simulink model "single_sat_attitude"  (R2018a)
settings: Solver=ode1  StartTime=0.0  StopTime=10.0  FixedStep=1/100  RelTol=1e-3
undefined symbols (not defined in the file or in its folder): Earth, h_init, hdmax, hmax, IAU, init, Kd, km, Kp, NRLMSISE_time_fromJD, q_init, s, wbn_init, WGS84
libraries: aerolibtransform2 x9, aerolibutil x6, sharedtransform x4, simulink x4, aerolibcelestial x3, vrlib x3, aerolibgravity2 x2, aerolibconvert2 x2, sharedutil x2, aerolibatmos2 x1
(part 2 of 2)

== system single_sat_attitude/Plant/Sun Torque and Force ==
  quat_in_body : Inport  PortDimensions=4
  sunBlocked : Inport  Port=2  OutDataTypeStr=boolean  PortDimensions=1
  sattosun_plant_eci : Inport  Port=3  PortDimensions=3
  4th real to 1st real : Subsystem
  Constant : Constant  Value=comtocops
  Constant1 : Constant  Value=unitnormals
  Constant2 : Constant  Value=areas
  Constant4 : Constant  Value=rss
  Constant5 : Constant  Value=rds
  Gain : Gain  Gain=-1
  Quaternion Rotation : aerolibutil/Quaternion Rotation
  Switch : Switch  Criteria=u2 ~= 0
  Zero : Constant  Value=0
  pressureTorque : MATLAB Function  TreatAsAtomicUnit=on
  solar pressure constant : Constant  Value=4.644E-6
  sunT_out_body : Outport  Unit=N*m  PortDimensions=3
  sunF_out_body : Outport  Port=2  Unit=N  PortDimensions=3
  wires:
  pressureTorque/2(torque) -> sunT_out_body/1
  Constant4/1 -> pressureTorque/6(rss)
  Constant/1 -> pressureTorque/5(comtocops)
  Constant1/1 -> pressureTorque/4(unitnormals)
  Constant2/1 -> pressureTorque/3(areas)
  sattosun_plant_eci/1 -> Quaternion Rotation/2
  Gain/1 -> pressureTorque/2(unitvelocity)
  Quaternion Rotation/1 -> Gain/1
  pressureTorque/1(force) -> sunF_out_body/1
  Constant5/1 -> pressureTorque/7(rds)
  sunBlocked/1 -> Switch/2
  Zero/1 -> Switch/1
  solar pressure constant/1 -> Switch/3
  Switch/1 -> pressureTorque/1(pressure)
  quat_in_body/1 -> 4th real to 1st real/1(qin)
  4th real to 1st real/1(qout) -> Quaternion Rotation/1

== system single_sat_attitude/Plant/circular_orbit ==
  time_elapsed : Inport  Unit=s  PortDimensions=1
  Gain1 : Gain  Gain=W
  Gain2 : Gain  Gain=PPERP
  Gain3 : Gain  Gain=P
  Gain4 : Gain  Gain=-P
  Gain5 : Gain  Gain=PPERP
  Gain6 : Gain  Gain=W
  Sin : Trigonometry
  Sin1 : Trigonometry  Operator=cos
  Sum2 : Sum  Inputs=+|+
  Sum5 : Sum  Inputs=+|+
  r_eci : Outport  Unit=m  PortDimensions=3
  v_eci : Outport  Port=2  Unit=m/s  PortDimensions=3
  wires:
  Gain5/1 -> Sum5/2
  Sum2/1 -> r_eci/1
  Gain2/1 -> Sum2/1
  Gain3/1 -> Sum2/2
  Gain4/1 -> Sum5/1
  Gain1/1 -> Sin/1, Sin1/1
  Sin1/1 -> Gain5/1, Gain3/1
  time_elapsed/1 -> Gain1/1
  Sum5/1 -> Gain6/1
  Sin/1 -> Gain4/1, Gain2/1
  Gain6/1 -> v_eci/1

== system single_sat_attitude/Sensor Model/Gyro ==
  note: Gyro: LSM6DS33
  body_w : Inport  Unit=rad/s
  DCM to translate from body to sensor : Constant  Value=init.IMU0_DCM_BODY
  Data Type Conversion : DataTypeConversion  OutDataTypeStr=int16  RndMeth=Round  SaturateOnIntegerOverflow=on
  Matrix Multiply1 : Product  Multiplication=Matrix(*)
  Random Number : RandomNumber  Mean=init.IMU0_G_TYOFF  Variance=init.IMU0_G_RMS.^2  SampleTime=1.0/init.IMU0_G_ODR
  Saturation : Saturate  UpperLimit=init.IMU0_G_FS  LowerLimit=-init.IMU0_G_FS
  Sum : Sum  Inputs=|++
  Zero-Order Hold : ZeroOrderHold  SampleTime=1.0/init.IMU0_G_ODR
  sensitivity : Gain  Gain=init.IMU0_G_GN
  sensor_w : Outport  OutDataTypeStr=int16
  wires:
  DCM to translate from body to sensor/1 -> Matrix Multiply1/1
  body_w/1 -> Matrix Multiply1/2
  sensitivity/1 -> Data Type Conversion/1
  Data Type Conversion/1 -> sensor_w/1
  Random Number/1 -> Sum/2
  Sum/1 -> sensitivity/1
  Saturation/1 -> Sum/1
  Zero-Order Hold/1 -> Saturation/1
  Matrix Multiply1/1 -> Zero-Order Hold/1

== system single_sat_attitude/Sensor Model/Magnetometer ==
  note: Magnetometer: LIS3MDL
      | see the data sheet for more details
  Magnetic_Field_body : Inport  Unit=nT
  DCM to translate from body to sensor : Constant  Value=init.IMU0_DCM_BODY
  Data Type Conversion : DataTypeConversion  OutDataTypeStr=int16  RndMeth=Round
  Matrix Multiply2 : Product  Multiplication=Matrix(*)
  Random Number : RandomNumber  Mean=-init.IMU0_MAG_ZGAUSS  Variance=init.IMU0_MAG_RMS.^2  SampleTime=1.0/init.IMU0_MAG_ODR
  Sum : Sum  Inputs=|++
  Zero-Order Hold : ZeroOrderHold  SampleTime=1.0/init.IMU0_MAG_ODR
  sensitivity : Gain  Gain=init.IMU0_MAG_GN
  Magxyz : Outport  OutDataTypeStr=int16
  wires:
  Data Type Conversion/1 -> Magxyz/1
  sensitivity/1 -> Data Type Conversion/1
  Matrix Multiply2/1 -> Zero-Order Hold/1
  Zero-Order Hold/1 -> Sum/1
  Sum/1 -> sensitivity/1
  Random Number/1 -> Sum/2
  Magnetic_Field_body/1 -> Matrix Multiply2/2
  DCM to translate from body to sensor/1 -> Matrix Multiply2/1

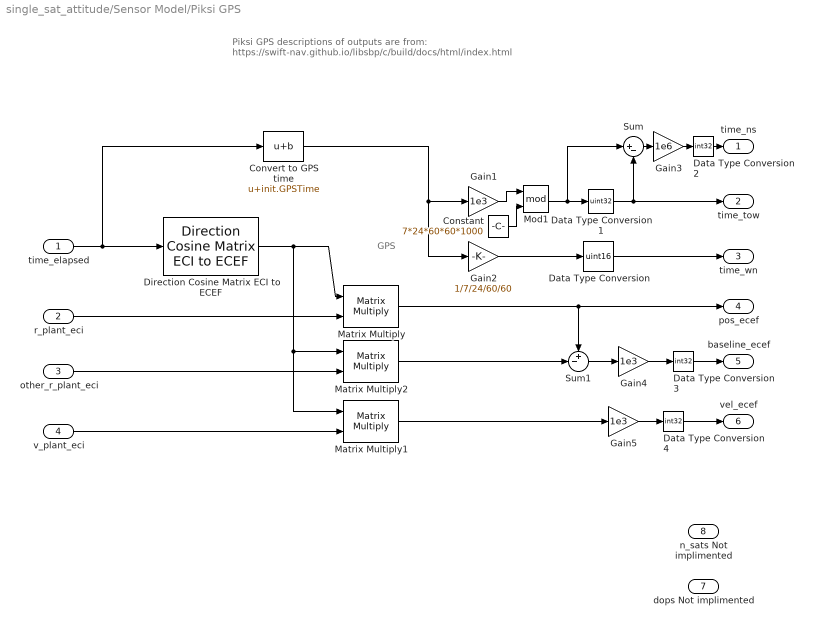
== system single_sat_attitude/Sensor Model/Piksi GPS ==
  note: Piksi GPS
      |
      | descriptions of outputs are from:
      | https://swift-nav.github.io/libsbp/c/build/docs/html/index.html
  note: GPS
  time_elapsed : Inport  Unit=s
  r_plant_eci : Inport  Port=2  Unit=m
  other_r_plant_eci : Inport  Port=3  Unit=m
  v_plant_eci : Inport  Port=4  Unit=m/s
  Constant : Constant  Value=7*24*60*60*1000
  Convert to GPS time : Bias  Bias=init.GPSTime
  Data Type Conversion : DataTypeConversion  OutDataTypeStr=uint16
  Data Type Conversion1 : DataTypeConversion  OutDataTypeStr=uint32  RndMeth=Round
  Data Type Conversion2 : DataTypeConversion  OutDataTypeStr=int32  RndMeth=Simplest
  Data Type Conversion3 : DataTypeConversion  OutDataTypeStr=int32  RndMeth=Simplest
  Data Type Conversion4 : DataTypeConversion  OutDataTypeStr=int32  RndMeth=Simplest
  Direction Cosine Matrix ECI to ECEF : aerolibtransform2/Direction Cosine Matrix ECI to ECEF  red=IAU-2000/2006  year=init.year  month=October  day=20  hour=init.hour  min=init.min  sec=init.sec  deltaT=Sec  errorflag=Error  extraparamflag=off
      settings: AttributesFormatString=%<red>  SourceProductName=Aerospace Blockset  SourceProductBaseCode=AE
  Gain1 : Gain  Gain=1e3
  Gain2 : Gain  Gain=1/7/24/60/60
  Gain3 : Gain  Gain=1e6
  Gain4 : Gain  Gain=1e3
  Gain5 : Gain  Gain=1e3
  Matrix Multiply : Product  Multiplication=Matrix(*)  OutDataTypeStr=double
  Matrix Multiply1 : Product  Multiplication=Matrix(*)
  Matrix Multiply2 : Product  Multiplication=Matrix(*)  OutDataTypeStr=double
  Mod1 : Math  Operator=mod  SaturateOnIntegerOverflow=on
  Sum : Sum  Inputs=|+-
  Sum1 : Sum  Inputs=+-|
  time_ns : Outport  OutMin=[-500000]  OutMax=[500000]  OutDataTypeStr=int32  Unit=ns  SampleTime=1/init.GPS_ODR
      settings: AttributesFormatString=Nanosecond residual of millisecond-rounded TOW
  time_tow : Outport  Port=2  OutMin=[0]  OutDataTypeStr=uint32  Unit=ms  SampleTime=1/init.GPS_ODR
      settings: AttributesFormatString=GPS time of week rounded to the nearest millisecond
  time_wn : Outport  Port=3  OutDataTypeStr=uint16  Unit=weeks  SampleTime=1/init.GPS_ODR
      settings: AttributesFormatString=GPS week number
  pos_ecef : Outport  Port=4  OutDataTypeStr=double  Unit=m  SampleTime=1/init.GPS_ODR
      settings: AttributesFormatString=absolute Earth Centered Earth Fixed (ECEF) coordinates
  baseline_ecef : Outport  Description=Dilution of Precision p,t  Port=5  OutDataTypeStr=int32  Unit=mm  SampleTime=1/init.GPS_ODR
      settings: AttributesFormatString=relative vector distance from the base station to the rover receiver.
  vel_ecef : Outport  Port=6  OutDataTypeStr=int32  Unit=mm/s  SampleTime=1/init.GPS_ODR
      settings: AttributesFormatString=velocity in Earth Centered Earth Fixed (ECEF) coordinates.
  dops Not implimented : Outport  Port=7  SampleTime=1/init.GPS_ODR
      settings: AttributesFormatString=|
      | Dilution of Precision p,t
      | describes the effect of navigation satellite geometry on positional measurement precision.
  n_sats Not implimented : Outport  Port=8  OutDataTypeStr=uint8  SampleTime=1/init.GPS_ODR
      settings: AttributesFormatString=Number of satellites used in solution.
  wires:
  Direction Cosine Matrix ECI to ECEF/1 -> Matrix Multiply1/1, Matrix Multiply2/1, Matrix Multiply/1
  time_elapsed/1 -> Direction Cosine Matrix ECI to ECEF/1, Convert to GPS time/1
  v_plant_eci/1 -> Matrix Multiply1/2
  Matrix Multiply/1 -> Sum1/1, pos_ecef/1
  r_plant_eci/1 -> Matrix Multiply/2
  Convert to GPS time/1 -> Gain2/1, Gain1/1
  Gain1/1 -> Mod1/1
  Data Type Conversion1/1 -> Sum/2, time_tow/1
  Sum/1 -> Gain3/1
  other_r_plant_eci/1 -> Matrix Multiply2/2
  Matrix Multiply2/1 -> Sum1/2
  Constant/1 -> Mod1/2
  Mod1/1 -> Data Type Conversion1/1, Sum/1
  Gain2/1 -> Data Type Conversion/1
  Data Type Conversion/1 -> time_wn/1
  Gain3/1 -> Data Type Conversion2/1
  Data Type Conversion2/1 -> time_ns/1
  Gain4/1 -> Data Type Conversion3/1
  Sum1/1 -> Gain4/1
  Data Type Conversion3/1 -> baseline_ecef/1
  Matrix Multiply1/1 -> Gain5/1
  Gain5/1 -> Data Type Conversion4/1
  Data Type Conversion4/1 -> vel_ecef/1

== system single_sat_attitude/Sensor Model/quat to DCM ==
  e0 e1 e2 e3 : Inport
  Demux : Demux
  Gain1 : Gain  Gain=2  SaturateOnIntegerOverflow=on  OutDataTypeStr=Inherit: Same as input  ParamDataTypeStr=Inherit: Same as input
  Gain2 : Gain  Gain=2  SaturateOnIntegerOverflow=on  OutDataTypeStr=Inherit: Same as input  ParamDataTypeStr=Inherit: Same as input
  Matrix Gain : Gain  Gain=eye(3,3)  SaturateOnIntegerOverflow=on  OutDataTypeStr=Inherit: Same as input  ParamDataTypeStr=Inherit: Same as input
  Mux : Mux  Inputs=3
  Product : Product  SaturateOnIntegerOverflow=on  InputSameDT=on  OutDataTypeStr=Inherit: Same as first input
  Product1 : Product  SaturateOnIntegerOverflow=on  InputSameDT=on  OutDataTypeStr=Inherit: Same as first input
  Subsystem : Subsystem
      mask Display: disp('3x3 cross matrix')
  Sum1 : Sum  Inputs=|+-  SaturateOnIntegerOverflow=on  InputSameDT=on  OutDataTypeStr=Inherit: Same as first input
  Sum8 : Sum  Inputs=|+-+  SaturateOnIntegerOverflow=on  InputSameDT=on  OutDataTypeStr=Inherit: Same as first input
  T1 : Math  Operator=transpose  SaturateOnIntegerOverflow=on
  T2 : Math  Operator=transpose  SaturateOnIntegerOverflow=on
  qTq : Product  Multiplication=Matrix(*)  SaturateOnIntegerOverflow=on  InputSameDT=on  OutDataTypeStr=Inherit: Same as first input
  qqT : Product  Multiplication=Matrix(*)  SaturateOnIntegerOverflow=on  InputSameDT=on  OutDataTypeStr=Inherit: Same as first input
  DCM : Outport  InitialOutput=0
  wires:
  Sum8/1 -> DCM/1
  e0 e1 e2 e3/1 -> Demux/1
  Demux/1 -> Mux/1
  Demux/2 -> Mux/2
  Demux/3 -> Mux/3
  Demux/4 -> Product/2, Product1/1, Product1/2
  Mux/1 -> T1/1, qqT/1, Subsystem/1(In1), T2/1, qTq/2
  Product/1 -> Gain1/1
  T1/1 -> qqT/2
  qqT/1 -> Gain2/1
  Gain2/1 -> Sum8/1
  Gain1/1 -> Sum8/2
  Product1/1 -> Sum1/1
  T2/1 -> qTq/1
  qTq/1 -> Sum1/2
  Sum1/1 -> Matrix Gain/1
  Matrix Gain/1 -> Sum8/3
  Subsystem/1(Out1) -> Product/1

== system single_sat_attitude/Actuator Model1/Rigid Body with Momentum Actuators and energy dissipation/Cross1 ==
  A : Inport  PortDimensions=3
  B : Inport  Port=2  PortDimensions=3
  Mux4 : Mux  Inputs=3
  Product{,1..5} (6 alike) : Product  SaturateOnIntegerOverflow=on  InputSameDT=on  OutDataTypeStr=Inherit: Same as first input
  Sum : Sum  Inputs=+-  SaturateOnIntegerOverflow=on  InputSameDT=on  OutDataTypeStr=Inherit: Same as first input
  Sum1 : Sum  Inputs=+-  SaturateOnIntegerOverflow=on  InputSameDT=on  OutDataTypeStr=Inherit: Same as first input
  Sum2 : Sum  Inputs=+-  SaturateOnIntegerOverflow=on  InputSameDT=on  OutDataTypeStr=Inherit: Same as first input
  demux2 : Demux  Outputs=3
  demux3 : Demux  Outputs=3
  AxB : Outport  InitialOutput=0
  wires:
  Mux4/1 -> AxB/1
  Sum2/1 -> Mux4/3
  Sum1/1 -> Mux4/2
  Sum/1 -> Mux4/1
  Product5/1 -> Sum2/2
  Product4/1 -> Sum2/1
  Product3/1 -> Sum1/2
  Product2/1 -> Sum1/1
  Product1/1 -> Sum/2
  Product/1 -> Sum/1
  demux3/1 -> Product5/2, Product2/2
  demux2/2 -> Product5/1, Product/1
  demux3/2 -> Product4/2, Product1/2
  demux2/1 -> Product4/1, Product3/1
  demux3/3 -> Product3/2, Product/2
  demux2/3 -> Product2/1, Product1/1
  B/1 -> demux3/1
  A/1 -> demux2/1

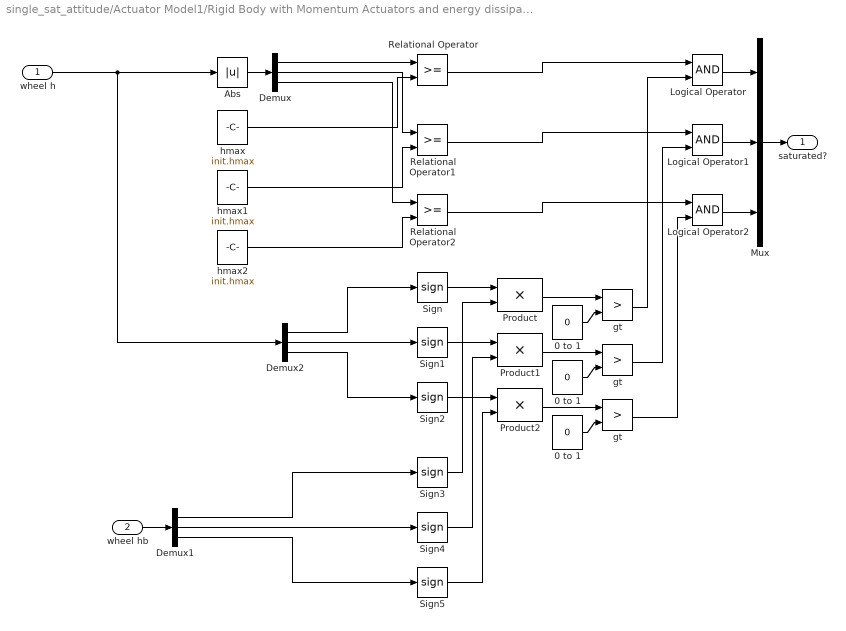
== system single_sat_attitude/Actuator Model1/Rigid Body with Momentum Actuators and energy dissipation/max rate check ==
  wheel h : Inport
  wheel hb : Inport  Port=2
  0 to 1 : Constant  Value=0  VectorParams1D=off
  "0 to 1 " : Constant  Value=0  VectorParams1D=off
  "0 to 1  " : Constant  Value=0  VectorParams1D=off
  Abs : Abs  SaturateOnIntegerOverflow=on
  Demux : Demux  Outputs=3
  Demux1 : Demux  Outputs=3
  Demux2 : Demux  Outputs=3
  Logical Operator : Logic
  Logical Operator1 : Logic
  Logical Operator2 : Logic
  Mux : Mux  Inputs=3
  Product : Product  SaturateOnIntegerOverflow=on  InputSameDT=on  OutDataTypeStr=Inherit: Same as first input
  Product1 : Product  SaturateOnIntegerOverflow=on  InputSameDT=on  OutDataTypeStr=Inherit: Same as first input
  Product2 : Product  SaturateOnIntegerOverflow=on  InputSameDT=on  OutDataTypeStr=Inherit: Same as first input
  Relational Operator : RelationalOperator  RndMeth=Nearest  InputSameDT=on
  Relational Operator1 : RelationalOperator  RndMeth=Nearest  InputSameDT=on
  Relational Operator2 : RelationalOperator  RndMeth=Nearest  InputSameDT=on
  Sign{,1..5} (6 alike) : Signum
  gt : RelationalOperator  Operator=>  RndMeth=Nearest  InputSameDT=on
  "gt " : RelationalOperator  Operator=>  RndMeth=Nearest  InputSameDT=on
  "gt  " : RelationalOperator  Operator=>  RndMeth=Nearest  InputSameDT=on
  hmax : Constant  Value=init.hmax  VectorParams1D=off
  hmax1 : Constant  Value=init.hmax  VectorParams1D=off
  hmax2 : Constant  Value=init.hmax  VectorParams1D=off
  saturated? : Outport
  wires:
  Abs/1 -> Demux/1
  Demux/1 -> Relational Operator/1
  Demux/2 -> Relational Operator1/1
  Demux/3 -> Relational Operator2/1
  hmax/1 -> Relational Operator/2
  hmax1/1 -> Relational Operator1/2
  hmax2/1 -> Relational Operator2/2
  wheel h/1 -> Abs/1, Demux2/1
  Mux/1 -> saturated?/1
  wheel hb/1 -> Demux1/1
  Demux1/1 -> Sign3/1
  Demux1/2 -> Sign4/1
  Demux1/3 -> Sign5/1
  Sign/1 -> Product/1
  Sign3/1 -> Product/2
  Sign1/1 -> Product1/1
  Sign4/1 -> Product1/2
  Sign2/1 -> Product2/1
  Sign5/1 -> Product2/2
  0 to 1/1 -> gt/2
  Product/1 -> gt/1
  "0 to 1 "/1 -> "gt "/2
  Product1/1 -> "gt "/1
  "0 to 1  "/1 -> "gt  "/2
  Product2/1 -> "gt  "/1
  Logical Operator/1 -> Mux/1
  Logical Operator1/1 -> Mux/2
  Logical Operator2/1 -> Mux/3
  Relational Operator/1 -> Logical Operator/1
  Relational Operator1/1 -> Logical Operator1/1
  Relational Operator2/1 -> Logical Operator2/1
  gt/1 -> Logical Operator/2
  "gt "/1 -> Logical Operator1/2
  "gt  "/1 -> Logical Operator2/2
  Demux2/1 -> Sign/1
  Demux2/2 -> Sign1/1
  Demux2/3 -> Sign2/1

== system single_sat_attitude/Actuator Model1/Rigid Body with Momentum Actuators and energy dissipation/quat to DCM ==
  e0 e1 e2 e3 : Inport
  Demux : Demux
  Gain1 : Gain  Gain=2  SaturateOnIntegerOverflow=on  OutDataTypeStr=Inherit: Same as input  ParamDataTypeStr=Inherit: Same as input
  Gain2 : Gain  Gain=2  SaturateOnIntegerOverflow=on  OutDataTypeStr=Inherit: Same as input  ParamDataTypeStr=Inherit: Same as input
  Matrix Gain : Gain  Gain=eye(3,3)  SaturateOnIntegerOverflow=on  OutDataTypeStr=Inherit: Same as input  ParamDataTypeStr=Inherit: Same as input
  Mux : Mux  Inputs=3
  Product : Product  SaturateOnIntegerOverflow=on  InputSameDT=on  OutDataTypeStr=Inherit: Same as first input
  Product1 : Product  SaturateOnIntegerOverflow=on  InputSameDT=on  OutDataTypeStr=Inherit: Same as first input
  Subsystem : Subsystem
      mask Display: disp('3x3 cross matrix')
  Sum1 : Sum  Inputs=|+-  SaturateOnIntegerOverflow=on  InputSameDT=on  OutDataTypeStr=Inherit: Same as first input
  Sum8 : Sum  Inputs=|+-+  SaturateOnIntegerOverflow=on  InputSameDT=on  OutDataTypeStr=Inherit: Same as first input
  T1 : Math  Operator=transpose  SaturateOnIntegerOverflow=on
  T2 : Math  Operator=transpose  SaturateOnIntegerOverflow=on
  qTq : Product  Multiplication=Matrix(*)  SaturateOnIntegerOverflow=on  InputSameDT=on  OutDataTypeStr=Inherit: Same as first input
  qqT : Product  Multiplication=Matrix(*)  SaturateOnIntegerOverflow=on  InputSameDT=on  OutDataTypeStr=Inherit: Same as first input
  DCM : Outport  InitialOutput=0
  wires:
  Subsystem/1(Out1) -> Product/1
  Matrix Gain/1 -> Sum8/3
  Sum1/1 -> Matrix Gain/1
  qTq/1 -> Sum1/2
  T2/1 -> qTq/1
  Product1/1 -> Sum1/1
  Gain1/1 -> Sum8/2
  Gain2/1 -> Sum8/1
  qqT/1 -> Gain2/1
  T1/1 -> qqT/2
  Product/1 -> Gain1/1
  Mux/1 -> qTq/2, T2/1, qqT/1, T1/1, Subsystem/1(In1)
  Demux/4 -> Product1/2, Product1/1, Product/2
  Demux/3 -> Mux/3
  Demux/2 -> Mux/2
  Demux/1 -> Mux/1
  e0 e1 e2 e3/1 -> Demux/1
  Sum8/1 -> DCM/1

== system single_sat_attitude/Actuator Model1/Rigid Body with Momentum Actuators and energy dissipation/quat to DCM1 ==
  e0 e1 e2 e3 : Inport
  Demux : Demux
  Gain1 : Gain  Gain=2  SaturateOnIntegerOverflow=on  OutDataTypeStr=Inherit: Same as input  ParamDataTypeStr=Inherit: Same as input
  Gain2 : Gain  Gain=2  SaturateOnIntegerOverflow=on  OutDataTypeStr=Inherit: Same as input  ParamDataTypeStr=Inherit: Same as input
  Matrix Gain : Gain  Gain=eye(3,3)  SaturateOnIntegerOverflow=on  OutDataTypeStr=Inherit: Same as input  ParamDataTypeStr=Inherit: Same as input
  Mux : Mux  Inputs=3
  Product : Product  SaturateOnIntegerOverflow=on  InputSameDT=on  OutDataTypeStr=Inherit: Same as first input
  Product1 : Product  SaturateOnIntegerOverflow=on  InputSameDT=on  OutDataTypeStr=Inherit: Same as first input
  Subsystem : Subsystem
      mask Display: disp('3x3 cross matrix')
  Sum1 : Sum  Inputs=|+-  SaturateOnIntegerOverflow=on  InputSameDT=on  OutDataTypeStr=Inherit: Same as first input
  Sum8 : Sum  Inputs=|+-+  SaturateOnIntegerOverflow=on  InputSameDT=on  OutDataTypeStr=Inherit: Same as first input
  T1 : Math  Operator=transpose  SaturateOnIntegerOverflow=on
  T2 : Math  Operator=transpose  SaturateOnIntegerOverflow=on
  qTq : Product  Multiplication=Matrix(*)  SaturateOnIntegerOverflow=on  InputSameDT=on  OutDataTypeStr=Inherit: Same as first input
  qqT : Product  Multiplication=Matrix(*)  SaturateOnIntegerOverflow=on  InputSameDT=on  OutDataTypeStr=Inherit: Same as first input
  DCM : Outport  InitialOutput=0
  wires:
  Subsystem/1(Out1) -> Product/1
  Matrix Gain/1 -> Sum8/3
  Sum1/1 -> Matrix Gain/1
  qTq/1 -> Sum1/2
  T2/1 -> qTq/1
  Product1/1 -> Sum1/1
  Gain1/1 -> Sum8/2
  Gain2/1 -> Sum8/1
  qqT/1 -> Gain2/1
  T1/1 -> qqT/2
  Product/1 -> Gain1/1
  Mux/1 -> qTq/2, T2/1, qqT/1, T1/1, Subsystem/1(In1)
  Demux/4 -> Product1/2, Product1/1, Product/2
  Demux/3 -> Mux/3
  Demux/2 -> Mux/2
  Demux/1 -> Mux/1
  e0 e1 e2 e3/1 -> Demux/1
  Sum8/1 -> DCM/1

== system single_sat_attitude/Attitude Determination/Attitude Determination/Generate reference vectors from Ephemeris and Magnetic Field Model ==
  note: geodetic LLA
  time_elapsed : Inport
  r_cs_sensor_eci : Inport  Port=2
  Add : Sum  Inputs=+-
  DecimalYearIncrement : Subsystem
  Demux : Demux  Outputs=3
  ECI Position to LLA : aerolibtransform2/ECI Position to LLA  red=IAU-2000/2006  year=init.year  month=October  day=20  hour=init.hour  min=init.min  sec=init.sec  deltaT=Sec  errorflag=Error  extraparamflag=off  eunits=Metric (MKS)  earthmodel=WGS84  flat=1/298.257223563  eqradius=6378137
      settings: AttributesFormatString=%<red>  SourceProductName=Aerospace Blockset  SourceProductBaseCode=AE
  International Geomagnetic Reference Field 12 : aerolibgravity2/International Geomagnetic Reference Field 12  units=Metric (MKS)  time_in=on  month=January  day=1  year=2020  action=None  sv_out=off
      settings: SourceProductName=Aerospace Blockset  SourceProductBaseCode=AE
  Julian Date : Subsystem
  Planetary Ephemeris : aerolibcelestial/Planetary Ephemeris  kmflag=km,km/s  epochflag=Julian date  de=DE430  nCenter=Earth  nTarget=Sun  errorflag=Error  velflag=off
      settings: SourceProductName=Aerospace Blockset  SourceProductBaseCode=AE
  r_Sun2cs_ref_eci : Outport
  r_MagField_ref_eci : Outport  Port=2
  wires:
  Julian Date/1(Julian Date) -> Planetary Ephemeris/1
  Planetary Ephemeris/1 -> Add/1
  Demux/1 -> International Geomagnetic Reference Field 12/2
  International Geomagnetic Reference Field 12/1 -> r_MagField_ref_eci/1
  ECI Position to LLA/1 -> Demux/1
  Demux/3 -> International Geomagnetic Reference Field 12/1
  Add/1 -> r_Sun2cs_ref_eci/1
  DecimalYearIncrement/1(DecimalYear) -> International Geomagnetic Reference Field 12/4
  r_cs_sensor_eci/1 -> Add/2, ECI Position to LLA/1
  time_elapsed/1 -> DecimalYearIncrement/1(clock_sec), ECI Position to LLA/2, Julian Date/1(deltaT)
  Demux/2 -> International Geomagnetic Reference Field 12/3

== system single_sat_attitude/Attitude Determination/Attitude Determination/Subsystem ==
  r_Sun2cs_ref_eci : Inport
  r_MagField_ref_eci : Inport  Port=2
  r_Sun2cs_sensor_body : Inport  Port=3
  r_MagField_sensor_body : Inport  Port=4
  MATLAB Function : MATLAB Function  TreatAsAtomicUnit=on
  quat_body_calc : Outport
  wires:
  r_Sun2cs_ref_eci/1 -> MATLAB Function/1(N_sun)
  r_MagField_ref_eci/1 -> MATLAB Function/2(N_mag)
  r_Sun2cs_sensor_body/1 -> MATLAB Function/3(B_sun)
  r_MagField_sensor_body/1 -> MATLAB Function/4(B_mag)
  MATLAB Function/1(q_triad) -> quat_body_calc/1

== system single_sat_attitude/Controller/Free Rigid Body with Momentum Actuators2/Cross ==
  A : Inport
  B : Inport  Port=2
  Mux4 : Mux  Inputs=3
  Product{,1..5} (6 alike) : Product  SaturateOnIntegerOverflow=on  InputSameDT=on  OutDataTypeStr=Inherit: Same as first input
  Sum : Sum  Inputs=+-  SaturateOnIntegerOverflow=on  InputSameDT=on  OutDataTypeStr=Inherit: Same as first input
  Sum1 : Sum  Inputs=+-  SaturateOnIntegerOverflow=on  InputSameDT=on  OutDataTypeStr=Inherit: Same as first input
  Sum2 : Sum  Inputs=+-  SaturateOnIntegerOverflow=on  InputSameDT=on  OutDataTypeStr=Inherit: Same as first input
  demux2 : Demux  Outputs=3
  demux3 : Demux  Outputs=3
  AxB : Outport  InitialOutput=0
  wires:
  Mux4/1 -> AxB/1
  Sum2/1 -> Mux4/3
  Sum1/1 -> Mux4/2
  Sum/1 -> Mux4/1
  Product5/1 -> Sum2/2
  Product4/1 -> Sum2/1
  Product3/1 -> Sum1/2
  Product2/1 -> Sum1/1
  Product1/1 -> Sum/2
  Product/1 -> Sum/1
  demux3/1 -> Product5/2, Product2/2
  demux2/2 -> Product5/1, Product/1
  demux3/2 -> Product4/2, Product1/2
  demux2/1 -> Product4/1, Product3/1
  demux3/3 -> Product3/2, Product/2
  demux2/3 -> Product2/1, Product1/1
  B/1 -> demux3/1
  A/1 -> demux2/1

== system single_sat_attitude/Controller/Free Rigid Body with Momentum Actuators2/Quaternion Integration ==
  w_Body : Inport
  Integrator1 : Integrator  InitialCondition=q_init
  q_normalize : Subsystem
  qderiv : Subsystem
  q_I_Body : Outport
  wires:
  qderiv/1(qd) -> Integrator1/1
  Integrator1/1 -> q_normalize/1(q_in)
  q_normalize/1(q_out) -> q_I_Body/1, qderiv/2(q)
  w_Body/1 -> qderiv/1(w)

== system single_sat_attitude/Controller/Free Rigid Body with Momentum Actuators2/RWA Saturation Model (Maxon EC 32 Flat 15W 24V) ==
  hb_com : Inport
  Demux : Demux  Outputs=3
  Demux2 : Demux  Outputs=3
  Max Torque : Saturate  UpperLimit=hdmax  LowerLimit=-hdmax
  Mux : Mux  Inputs=3
  Scope : Scope
  Switch : Switch  Threshold=0.5  SaturateOnIntegerOverflow=on  InputSameDT=on
  Switch1 : Switch  Threshold=0.5  SaturateOnIntegerOverflow=on  InputSameDT=on
  Switch2 : Switch  Threshold=0.5  SaturateOnIntegerOverflow=on  InputSameDT=on
  "hb -> h" : Integrator  InitialCondition=h_init
  max rate check : Subsystem
  no torque : Constant  Value=0
  hb_act : Outport
  h_act : Outport  Port=2
  wires:
  Switch2/1 -> Mux/3
  Switch1/1 -> Mux/2
  Demux2/3 -> Switch2/2
  Switch/1 -> Mux/1
  no torque/1 -> Switch/1, Switch1/1, Switch2/1
  Demux2/1 -> Switch/2
  Mux/1 -> Scope/1, hb_act/1, "hb -> h"/1
  hb_com/1 -> Max Torque/1
  Demux2/2 -> Switch1/2
  Demux/2 -> Switch1/3
  Demux/1 -> Switch/3
  "hb -> h"/1 -> h_act/1, max rate check/1(wheel h)
  Max Torque/1 -> Demux/1, max rate check/2(wheel hb)
  Demux/3 -> Switch2/3
  max rate check/1(saturated?) -> Demux2/1

== system single_sat_attitude/Controller/Free Rigid Body with Momentum Actuators2/compute attitude error ==
  quat : Inport
  quat_cmd : Inport  Port=2
  Demux : Demux
  Mux : Mux  Inputs=3
  Mux1 : Mux  Inputs=2
  quat_multiply (relative quat) : Subsystem
  reverse : Gain  Gain=-1  SaturateOnIntegerOverflow=on  OutDataTypeStr=Inherit: Same as input  ParamDataTypeStr=Inherit: Same as input
  quat error : Outport
  wires:
  quat/1 -> quat_multiply (relative quat)/1(q_bc)
  quat_cmd/1 -> Demux/1
  Demux/1 -> Mux/1
  Demux/2 -> Mux/2
  Demux/3 -> Mux/3
  Demux/4 -> reverse/1
  Mux/1 -> Mux1/1
  Mux1/1 -> quat_multiply (relative quat)/2(q_ab)
  reverse/1 -> Mux1/2
  quat_multiply (relative quat)/1(q_ac) -> quat error/1

== system single_sat_attitude/Controller/Normal Mode Control System/Cross3 ==
  A : Inport
  B : Inport  Port=2
  Mux4 : Mux  Inputs=3
  Product{,1..5} (6 alike) : Product  SaturateOnIntegerOverflow=on  InputSameDT=on  OutDataTypeStr=Inherit: Same as first input
  Sum : Sum  Inputs=+-  SaturateOnIntegerOverflow=on  InputSameDT=on  OutDataTypeStr=Inherit: Same as first input
  Sum1 : Sum  Inputs=+-  SaturateOnIntegerOverflow=on  InputSameDT=on  OutDataTypeStr=Inherit: Same as first input
  Sum2 : Sum  Inputs=+-  SaturateOnIntegerOverflow=on  InputSameDT=on  OutDataTypeStr=Inherit: Same as first input
  demux2 : Demux  Outputs=3
  demux3 : Demux  Outputs=3
  AxB : Outport  InitialOutput=0
  wires:
  A/1 -> demux2/1
  B/1 -> demux3/1
  demux2/3 -> Product1/1, Product2/1
  demux3/3 -> Product/2, Product3/2
  demux2/1 -> Product3/1, Product4/1
  demux3/2 -> Product1/2, Product4/2
  demux2/2 -> Product/1, Product5/1
  demux3/1 -> Product2/2, Product5/2
  Product/1 -> Sum/1
  Product1/1 -> Sum/2
  Product2/1 -> Sum1/1
  Product3/1 -> Sum1/2
  Product4/1 -> Sum2/1
  Product5/1 -> Sum2/2
  Sum/1 -> Mux4/1
  Sum1/1 -> Mux4/2
  Sum2/1 -> Mux4/3
  Mux4/1 -> AxB/1

== system single_sat_attitude/Controller/Normal Mode Control System/Magnet Torquer ==
  m_mt_des : Inport
  Abs : Abs  SaturateOnIntegerOverflow=on
  Constant : Constant  Value=0
  Demux : Demux  Outputs=3
  Demux1 : Demux  Outputs=3
  Mux : Mux  Inputs=3
  Relational Operator1 : RelationalOperator  Operator===  RndMeth=Nearest  InputSameDT=on
  Relational Operator2 : RelationalOperator  Operator===  RndMeth=Nearest  InputSameDT=on
  Relational Operator3 : RelationalOperator  Operator===  RndMeth=Nearest  InputSameDT=on
  Switch1 : Switch  Threshold=0.5  SaturateOnIntegerOverflow=on  InputSameDT=on
  Switch2 : Switch  Threshold=0.5  SaturateOnIntegerOverflow=on  InputSameDT=on
  Switch3 : Switch  Threshold=0.5  SaturateOnIntegerOverflow=on  InputSameDT=on
  m_mt : Constant  Value=init.m_mt  VectorParams1D=off
  m_mt1 : Constant  Value=init.m_mt  VectorParams1D=off
  m_mt2 : Constant  Value=init.m_mt  VectorParams1D=off
  m_mt_cmd : Outport
  wires:
  Mux/1 -> m_mt_cmd/1
  Abs/1 -> Demux/1
  m_mt/1 -> Relational Operator1/2
  Demux/1 -> Relational Operator1/1
  m_mt1/1 -> Relational Operator2/2
  m_mt2/1 -> Relational Operator3/2
  Demux/2 -> Relational Operator2/1
  Demux/3 -> Relational Operator3/1
  Relational Operator1/1 -> Switch1/2
  Relational Operator2/1 -> Switch2/2
  Relational Operator3/1 -> Switch3/2
  Demux1/1 -> Switch1/1
  Demux1/3 -> Switch3/1
  Demux1/2 -> Switch2/1
  m_mt_des/1 -> Demux1/1, Abs/1
  Constant/1 -> Switch3/3, Switch2/3, Switch1/3
  Switch1/1 -> Mux/1
  Switch2/1 -> Mux/2
  Switch3/1 -> Mux/3

== system single_sat_attitude/Controller/Normal Mode Control System/compute attitude error ==
  quat : Inport
  quat_cmd : Inport  Port=2
  Demux : Demux
  Demux1 : Demux
  Mux : Mux  Inputs=3
  Mux1 : Mux  Inputs=2
  Mux2 : Mux  Inputs=3
  Mux3 : Mux  Inputs=2
  Selector : Selector  InputPortWidth=4  IndexOptions=Index vector (dialog)  Indices=4  OutputSizes=1
  Switch : Switch
  quat_multiply (relative quat) : Subsystem
  quat_multiply (relative quat)1 : Subsystem
  reverse : Gain  Gain=-1  SaturateOnIntegerOverflow=on  OutDataTypeStr=Inherit: Same as input  ParamDataTypeStr=Inherit: Same as input
  reverse1 : Gain  Gain=-1  SaturateOnIntegerOverflow=on  OutDataTypeStr=Inherit: Same as input  ParamDataTypeStr=Inherit: Same as input
  quat error : Outport
  wires:
  Demux/1 -> Mux/1
  Demux/2 -> Mux/2
  Demux/3 -> Mux/3
  Mux/1 -> reverse/1
  Mux1/1 -> quat_multiply (relative quat)/2(q_ab)
  Demux/4 -> Mux1/2
  reverse/1 -> Mux1/1
  Mux3/1 -> quat_multiply (relative quat)1/2(q_ab)
  Demux1/1 -> Mux2/1
  Demux1/2 -> Mux2/2
  Demux1/3 -> Mux2/3
  quat_cmd/1 -> Demux1/1, Demux/1
  Mux2/1 -> Mux3/1
  quat/1 -> quat_multiply (relative quat)1/1(q_bc), quat_multiply (relative quat)/1(q_bc)
  Demux1/4 -> reverse1/1
  reverse1/1 -> Mux3/2
  quat_multiply (relative quat)1/1(q_ac) -> Switch/3
  quat_multiply (relative quat)/1(q_ac) -> Selector/1, Switch/1
  Switch/1 -> quat error/1
  Selector/1 -> Switch/2

== system single_sat_attitude/Plant/Atm Torque and Force/4th real to 1st real ==
  qin : Inport
  Demux : Demux
  Mux : Mux
  qout : Outport
  wires:
  qin/1 -> Demux/1
  Demux/4 -> Mux/1
  Demux/1 -> Mux/2
  Demux/2 -> Mux/3
  Demux/3 -> Mux/4
  Mux/1 -> qout/1

== system single_sat_attitude/Plant/Grav Torque/4th real to 1st real ==
  qin : Inport
  Demux : Demux
  Mux : Mux
  qout : Outport
  wires:
  qin/1 -> Demux/1
  Demux/4 -> Mux/1
  Demux/1 -> Mux/2
  Demux/2 -> Mux/3
  Demux/3 -> Mux/4
  Mux/1 -> qout/1

== system single_sat_attitude/Plant/Quaternion Integration/q_normalize ==
  q_in : Inport  PortDimensions=4
  Dot Product : DotProduct  InputSameDT=on  OutDataTypeStr=Inherit: Inherit via internal rule
  Math Function : Math  Operator=sqrt  SaturateOnIntegerOverflow=on
  Product : Product  Inputs=*/  SaturateOnIntegerOverflow=on  InputSameDT=on  OutDataTypeStr=Inherit: Same as first input
  q_out : Outport
  wires:
  q_in/1 -> Dot Product/1, Dot Product/2, Product/1
  Dot Product/1 -> Math Function/1
  Math Function/1 -> Product/2
  Product/1 -> q_out/1

== system single_sat_attitude/Plant/Quaternion Integration/qderiv ==
  w : Inport
  q : Inport  Port=2
  Mux : Mux  Inputs=2
  Mux1 : Mux
  qd1 : Fcn  Expr=(u(7)*u(1)-u(6)*u(2)+u(5)*u(3))/2
  qd2 : Fcn  Expr=(u(6)*u(1)+u(7)*u(2)-u(4)*u(3))/2
  qd3 : Fcn  Expr=(-u(5)*u(1)+u(4)*u(2)+u(7)*u(3))/2
  qd4 : Fcn  Expr=(-u(4)*u(1)-u(5)*u(2)-u(6)*u(3))/2
  qd : Outport
  wires:
  w/1 -> Mux/1
  q/1 -> Mux/2
  Mux/1 -> qd3/1, qd4/1, qd1/1, qd2/1
  qd1/1 -> Mux1/1
  qd2/1 -> Mux1/2
  qd3/1 -> Mux1/3
  qd4/1 -> Mux1/4
  Mux1/1 -> qd/1

== system single_sat_attitude/Plant/Sun Torque and Force/4th real to 1st real ==
  qin : Inport
  Demux : Demux
  Mux : Mux
  qout : Outport
  wires:
  qin/1 -> Demux/1
  Demux/4 -> Mux/1
  Demux/1 -> Mux/2
  Demux/2 -> Mux/3
  Demux/3 -> Mux/4
  Mux/1 -> qout/1

== system single_sat_attitude/Sensor Model/quat to DCM/Subsystem ==
  In1 : Inport
  3x3 : Reshape  OutputDimensionality=Customize  OutputDimensions=[3,3]
  Demux : Demux  Outputs=3
  Gain : Gain  Gain=-1  SaturateOnIntegerOverflow=on  OutDataTypeStr=Inherit: Same as input  ParamDataTypeStr=Inherit: Same as input
  Gain1 : Gain  Gain=-1  SaturateOnIntegerOverflow=on  OutDataTypeStr=Inherit: Same as input  ParamDataTypeStr=Inherit: Same as input
  Gain2 : Gain  Gain=-1  SaturateOnIntegerOverflow=on  OutDataTypeStr=Inherit: Same as input  ParamDataTypeStr=Inherit: Same as input
  Mux : Mux  Inputs=9
  "diag 0 " : Constant  Value=0
  Out1 : Outport
  wires:
  In1/1 -> Demux/1
  3x3/1 -> Out1/1
  "diag 0 "/1 -> Mux/1, Mux/5, Mux/9
  Mux/1 -> 3x3/1
  Demux/3 -> Mux/2, Gain1/1
  Gain/1 -> Mux/3
  Demux/2 -> Gain/1, Mux/7
  Gain1/1 -> Mux/4
  Demux/1 -> Mux/6, Gain2/1
  Gain2/1 -> Mux/8

== system single_sat_attitude/Actuator Model1/Rigid Body with Momentum Actuators and energy dissipation/quat to DCM/Subsystem ==
  In1 : Inport
  3x3 : Reshape  OutputDimensionality=Customize  OutputDimensions=[3,3]
  Demux : Demux  Outputs=3
  Gain : Gain  Gain=-1  SaturateOnIntegerOverflow=on  OutDataTypeStr=Inherit: Same as input  ParamDataTypeStr=Inherit: Same as input
  Gain1 : Gain  Gain=-1  SaturateOnIntegerOverflow=on  OutDataTypeStr=Inherit: Same as input  ParamDataTypeStr=Inherit: Same as input
  Gain2 : Gain  Gain=-1  SaturateOnIntegerOverflow=on  OutDataTypeStr=Inherit: Same as input  ParamDataTypeStr=Inherit: Same as input
  Mux : Mux  Inputs=9
  "diag 0 " : Constant  Value=0
  Out1 : Outport
  wires:
  Gain2/1 -> Mux/8
  Demux/1 -> Gain2/1, Mux/6
  Gain1/1 -> Mux/4
  Demux/2 -> Mux/7, Gain/1
  Gain/1 -> Mux/3
  Demux/3 -> Gain1/1, Mux/2
  Mux/1 -> 3x3/1
  "diag 0 "/1 -> Mux/9, Mux/5, Mux/1
  3x3/1 -> Out1/1
  In1/1 -> Demux/1

== system single_sat_attitude/Actuator Model1/Rigid Body with Momentum Actuators and energy dissipation/quat to DCM1/Subsystem ==
  In1 : Inport
  3x3 : Reshape  OutputDimensionality=Customize  OutputDimensions=[3,3]
  Demux : Demux  Outputs=3
  Gain : Gain  Gain=-1  SaturateOnIntegerOverflow=on  OutDataTypeStr=Inherit: Same as input  ParamDataTypeStr=Inherit: Same as input
  Gain1 : Gain  Gain=-1  SaturateOnIntegerOverflow=on  OutDataTypeStr=Inherit: Same as input  ParamDataTypeStr=Inherit: Same as input
  Gain2 : Gain  Gain=-1  SaturateOnIntegerOverflow=on  OutDataTypeStr=Inherit: Same as input  ParamDataTypeStr=Inherit: Same as input
  Mux : Mux  Inputs=9
  "diag 0 " : Constant  Value=0
  Out1 : Outport
  wires:
  Gain2/1 -> Mux/8
  Demux/1 -> Gain2/1, Mux/6
  Gain1/1 -> Mux/4
  Demux/2 -> Mux/7, Gain/1
  Gain/1 -> Mux/3
  Demux/3 -> Gain1/1, Mux/2
  Mux/1 -> 3x3/1
  "diag 0 "/1 -> Mux/9, Mux/5, Mux/1
  3x3/1 -> Out1/1
  In1/1 -> Demux/1

== system single_sat_attitude/Attitude Determination/Attitude Determination/Generate reference vectors from Ephemeris and Magnetic Field Model/DecimalYearIncrement ==
  note: day
  clock_sec : Inport
  Add : Sum
  Constant : Constant  Value=init.year
  Constant1 : Constant  Value=init.month
  Constant2 : Constant  Value=init.day
  Constant3 : Constant  Value=init.hour
  Constant4 : Constant  Value=init.min
  Constant5 : Constant  Value=init.min
  Divide : Product  Inputs=*/
  MATLAB Function : MATLAB Function  TreatAsAtomicUnit=on
  Product2 : Product  Inputs=*/
  day2decimalYear : Constant  Value=365
  sec2day : Constant  Value=86400
  DecimalYear : Outport
  wires:
  Product2/1 -> Divide/1
  sec2day/1 -> Product2/2
  Add/1 -> DecimalYear/1
  Constant3/1 -> MATLAB Function/4(hour)
  day2decimalYear/1 -> Divide/2
  Divide/1 -> Add/1
  MATLAB Function/1(DecimalYear) -> Add/2
  Constant1/1 -> MATLAB Function/2(month)
  Constant/1 -> MATLAB Function/1(year)
  Constant4/1 -> MATLAB Function/5(minute)
  Constant5/1 -> MATLAB Function/6(second)
  clock_sec/1 -> Product2/1
  Constant2/1 -> MATLAB Function/3(day)

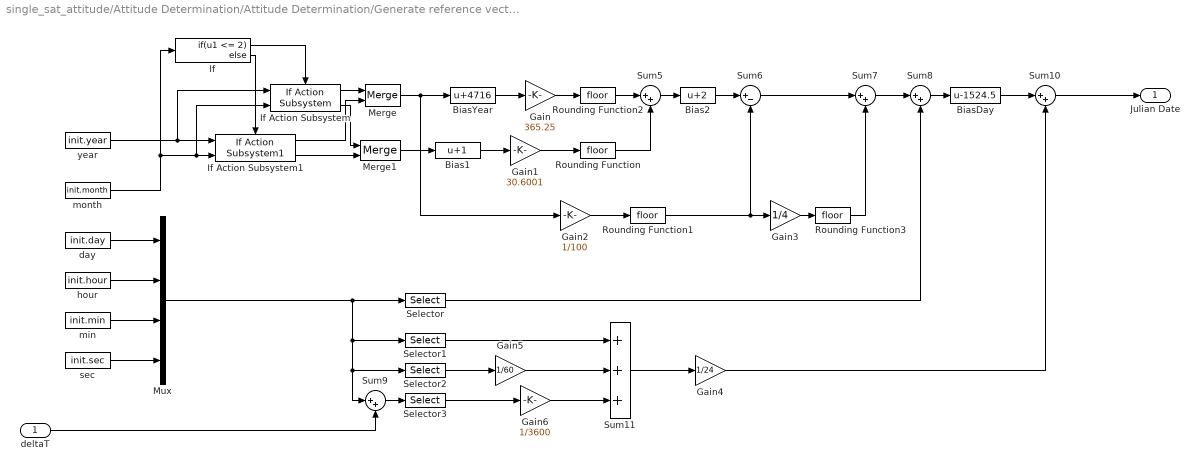
== system single_sat_attitude/Attitude Determination/Attitude Determination/Generate reference vectors from Ephemeris and Magnetic Field Model/Julian Date ==
  deltaT : Inport  OutMin=0  PortDimensions=1
  Bias1 : Bias  Bias=1
  Bias2 : Bias  Bias=2
  BiasDay : Bias  Bias=-1524.5
  BiasYear : Bias  Bias=4716
  Gain : Gain  Gain=365.25
  Gain1 : Gain  Gain=30.6001
  Gain2 : Gain  Gain=1/100
  Gain3 : Gain  Gain=1/4
  Gain4 : Gain  Gain=1/24
  Gain5 : Gain  Gain=1/60
  Gain6 : Gain  Gain=1/3600
  If : If  IfExpression=u1 <= 2
  If Action Subsystem : aerolibconvert2/Julian Date Conversion/If Action Subsystem
      settings: SourceProductName=Aerospace Blockset  SourceProductBaseCode=AE
  If Action Subsystem1 : aerolibconvert2/Julian Date Conversion/If Action Subsystem1
      settings: SourceProductName=Aerospace Blockset  SourceProductBaseCode=AE
  Merge : Merge
  Merge1 : Merge
  Mux : Mux
  Rounding Function{,1..3} (4 alike) : Rounding
  Selector : Selector  InputPortWidth=4  IndexOptions=Index vector (dialog)  Indices=[1]  OutputSizes=1
  Selector1 : Selector  InputPortWidth=4  IndexOptions=Index vector (dialog)  Indices=[2]  OutputSizes=1
  Selector2 : Selector  InputPortWidth=4  IndexOptions=Index vector (dialog)  Indices=[3]  OutputSizes=1
  Selector3 : Selector  InputPortWidth=4  IndexOptions=Index vector (dialog)  Indices=[4]  OutputSizes=1
  Sum{5,7..10} (5 alike) : Sum  Inputs=|++
  Sum11 : Sum  Inputs=+++
  Sum6 : Sum  Inputs=|+-
  day : Constant  Value=init.day
  hour : Constant  Value=init.hour
  min : Constant  Value=init.min
  month : Constant  Value=init.month
  sec : Constant  Value=init.sec
  year : Constant  Value=init.year
  Julian Date : Outport
  wires:
  If Action Subsystem/1 -> Merge/1
  If/2 -> If Action Subsystem1/Action
  year/1 -> If Action Subsystem/1, If Action Subsystem1/1
  If/1 -> If Action Subsystem/Action
  If Action Subsystem/2 -> Merge1/1
  Rounding Function3/1 -> Sum7/2
  deltaT/1 -> Sum9/2
  day/1 -> Mux/1
  Merge1/1 -> Bias1/1
  Gain/1 -> Rounding Function2/1
  Gain2/1 -> Rounding Function1/1
  Merge/1 -> Gain2/1, BiasYear/1
  Selector3/1 -> Gain6/1
  Sum6/1 -> Sum7/1
  Gain5/1 -> Sum11/2
  BiasYear/1 -> Gain/1
  Selector2/1 -> Gain5/1
  Gain6/1 -> Sum11/3
  Sum11/1 -> Gain4/1
  Gain3/1 -> Rounding Function3/1
  Selector1/1 -> Sum11/1
  If Action Subsystem1/1 -> Merge/2
  Sum7/1 -> Sum8/1
  Mux/1 -> Selector1/1, Sum9/1, Selector2/1, Selector/1
  Sum10/1 -> Julian Date/1
  Selector/1 -> Sum8/2
  Bias1/1 -> Gain1/1
  sec/1 -> Mux/4
  If Action Subsystem1/2 -> Merge1/2
  Sum5/1 -> Bias2/1
  BiasDay/1 -> Sum10/1
  Gain1/1 -> Rounding Function/1
  Rounding Function1/1 -> Gain3/1, Sum6/2
  Bias2/1 -> Sum6/1
  Sum8/1 -> BiasDay/1
  Rounding Function2/1 -> Sum5/1
  Rounding Function/1 -> Sum5/2
  month/1 -> If Action Subsystem/2, If Action Subsystem1/2, If/1
  min/1 -> Mux/3
  hour/1 -> Mux/2
  Gain4/1 -> Sum10/2
  Sum9/1 -> Selector3/1

== system single_sat_attitude/Controller/Free Rigid Body with Momentum Actuators2/Quaternion Integration/q_normalize ==
  q_in : Inport  PortDimensions=4
  Dot Product : DotProduct  InputSameDT=on  OutDataTypeStr=Inherit: Inherit via internal rule
  Math Function : Math  Operator=sqrt  SaturateOnIntegerOverflow=on
  Product : Product  Inputs=*/  SaturateOnIntegerOverflow=on  InputSameDT=on  OutDataTypeStr=Inherit: Same as first input
  q_out : Outport
  wires:
  q_in/1 -> Dot Product/1, Dot Product/2, Product/1
  Dot Product/1 -> Math Function/1
  Math Function/1 -> Product/2
  Product/1 -> q_out/1

== system single_sat_attitude/Controller/Free Rigid Body with Momentum Actuators2/Quaternion Integration/qderiv ==
  w : Inport
  q : Inport  Port=2
  Mux : Mux  Inputs=2
  Mux1 : Mux
  qd1 : Fcn  Expr=(u(7)*u(1)-u(6)*u(2)+u(5)*u(3))/2
  qd2 : Fcn  Expr=(u(6)*u(1)+u(7)*u(2)-u(4)*u(3))/2
  qd3 : Fcn  Expr=(-u(5)*u(1)+u(4)*u(2)+u(7)*u(3))/2
  qd4 : Fcn  Expr=(-u(4)*u(1)-u(5)*u(2)-u(6)*u(3))/2
  qd : Outport
  wires:
  w/1 -> Mux/1
  q/1 -> Mux/2
  Mux/1 -> qd3/1, qd4/1, qd1/1, qd2/1
  qd1/1 -> Mux1/1
  qd2/1 -> Mux1/2
  qd3/1 -> Mux1/3
  qd4/1 -> Mux1/4
  Mux1/1 -> qd/1

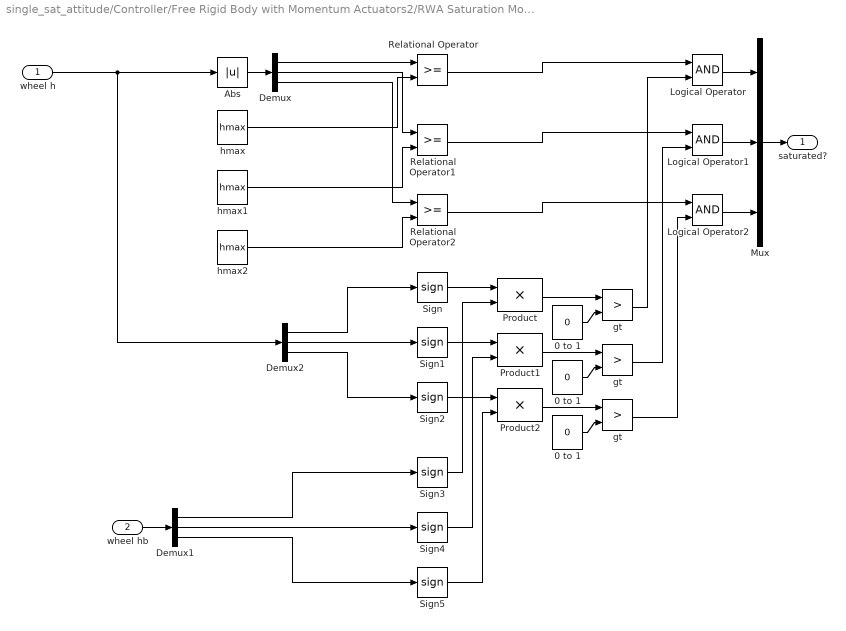
== system single_sat_attitude/Controller/Free Rigid Body with Momentum Actuators2/RWA Saturation Model (Maxon EC 32 Flat 15W 24V)/max rate check ==
  wheel h : Inport
  wheel hb : Inport  Port=2
  0 to 1 : Constant  Value=0  VectorParams1D=off
  "0 to 1 " : Constant  Value=0  VectorParams1D=off
  "0 to 1  " : Constant  Value=0  VectorParams1D=off
  Abs : Abs  SaturateOnIntegerOverflow=on
  Demux : Demux  Outputs=3
  Demux1 : Demux  Outputs=3
  Demux2 : Demux  Outputs=3
  Logical Operator : Logic
  Logical Operator1 : Logic
  Logical Operator2 : Logic
  Mux : Mux  Inputs=3
  Product : Product  SaturateOnIntegerOverflow=on  InputSameDT=on  OutDataTypeStr=Inherit: Same as first input
  Product1 : Product  SaturateOnIntegerOverflow=on  InputSameDT=on  OutDataTypeStr=Inherit: Same as first input
  Product2 : Product  SaturateOnIntegerOverflow=on  InputSameDT=on  OutDataTypeStr=Inherit: Same as first input
  Relational Operator : RelationalOperator  RndMeth=Nearest  InputSameDT=on
  Relational Operator1 : RelationalOperator  RndMeth=Nearest  InputSameDT=on
  Relational Operator2 : RelationalOperator  RndMeth=Nearest  InputSameDT=on
  Sign{,1..5} (6 alike) : Signum
  gt : RelationalOperator  Operator=>  RndMeth=Nearest  InputSameDT=on
  "gt " : RelationalOperator  Operator=>  RndMeth=Nearest  InputSameDT=on
  "gt  " : RelationalOperator  Operator=>  RndMeth=Nearest  InputSameDT=on
  hmax : Constant  Value=hmax  VectorParams1D=off
  hmax1 : Constant  Value=hmax  VectorParams1D=off
  hmax2 : Constant  Value=hmax  VectorParams1D=off
  saturated? : Outport
  wires:
  Abs/1 -> Demux/1
  Demux/1 -> Relational Operator/1
  Demux/2 -> Relational Operator1/1
  Demux/3 -> Relational Operator2/1
  hmax/1 -> Relational Operator/2
  hmax1/1 -> Relational Operator1/2
  hmax2/1 -> Relational Operator2/2
  wheel h/1 -> Abs/1, Demux2/1
  Mux/1 -> saturated?/1
  wheel hb/1 -> Demux1/1
  Demux1/1 -> Sign3/1
  Demux1/2 -> Sign4/1
  Demux1/3 -> Sign5/1
  Sign/1 -> Product/1
  Sign3/1 -> Product/2
  Sign1/1 -> Product1/1
  Sign4/1 -> Product1/2
  Sign2/1 -> Product2/1
  Sign5/1 -> Product2/2
  0 to 1/1 -> gt/2
  Product/1 -> gt/1
  "0 to 1 "/1 -> "gt "/2
  Product1/1 -> "gt "/1
  "0 to 1  "/1 -> "gt  "/2
  Product2/1 -> "gt  "/1
  Logical Operator/1 -> Mux/1
  Logical Operator1/1 -> Mux/2
  Logical Operator2/1 -> Mux/3
  Relational Operator/1 -> Logical Operator/1
  Relational Operator1/1 -> Logical Operator1/1
  Relational Operator2/1 -> Logical Operator2/1
  gt/1 -> Logical Operator/2
  "gt "/1 -> Logical Operator1/2
  "gt  "/1 -> Logical Operator2/2
  Demux2/1 -> Sign/1
  Demux2/2 -> Sign1/1
  Demux2/3 -> Sign2/1

== system single_sat_attitude/Controller/Free Rigid Body with Momentum Actuators2/compute attitude error/quat_multiply (relative quat) ==
  q_bc : Inport
  q_ab : Inport  Port=2
  Mux : Mux  Inputs=2
  Mux1 : Mux
  qerr1 : Fcn  Expr=u(4)*u(5)+u(3)*u(6)-u(2)*u(7)+u(1)*u(8)
  qerr2 : Fcn  Expr=-u(3)*u(5)+u(4)*u(6)+u(1)*u(7)+u(2)*u(8)
  qerr3 : Fcn  Expr=u(2)*u(5)-u(1)*u(6)+u(4)*u(7)+u(3)*u(8)
  qerr4 : Fcn  Expr=-u(1)*u(5)-u(2)*u(6)-u(3)*u(7)+u(4)*u(8)
  q_ac : Outport
  wires:
  Mux1/1 -> q_ac/1
  qerr4/1 -> Mux1/4
  qerr3/1 -> Mux1/3
  qerr2/1 -> Mux1/2
  qerr1/1 -> Mux1/1
  Mux/1 -> qerr4/1, qerr3/1, qerr2/1, qerr1/1
  q_ab/1 -> Mux/2
  q_bc/1 -> Mux/1

== system single_sat_attitude/Controller/Normal Mode Control System/compute attitude error/quat_multiply (relative quat) ==
  q_bc : Inport
  q_ab : Inport  Port=2
  Mux : Mux  Inputs=2
  Mux1 : Mux
  qerr1 : Fcn  Expr=u(4)*u(5)+u(3)*u(6)-u(2)*u(7)+u(1)*u(8)
  qerr2 : Fcn  Expr=-u(3)*u(5)+u(4)*u(6)+u(1)*u(7)+u(2)*u(8)
  qerr3 : Fcn  Expr=u(2)*u(5)-u(1)*u(6)+u(4)*u(7)+u(3)*u(8)
  qerr4 : Fcn  Expr=-u(1)*u(5)-u(2)*u(6)-u(3)*u(7)+u(4)*u(8)
  q_ac : Outport
  wires:
  Mux1/1 -> q_ac/1
  qerr4/1 -> Mux1/4
  qerr3/1 -> Mux1/3
  qerr2/1 -> Mux1/2
  qerr1/1 -> Mux1/1
  Mux/1 -> qerr4/1, qerr3/1, qerr2/1, qerr1/1
  q_ab/1 -> Mux/2
  q_bc/1 -> Mux/1

== system single_sat_attitude/Controller/Normal Mode Control System/compute attitude error/quat_multiply (relative quat)1 ==
  q_bc : Inport
  q_ab : Inport  Port=2
  Mux : Mux  Inputs=2
  Mux1 : Mux
  qerr1 : Fcn  Expr=u(4)*u(5)+u(3)*u(6)-u(2)*u(7)+u(1)*u(8)
  qerr2 : Fcn  Expr=-u(3)*u(5)+u(4)*u(6)+u(1)*u(7)+u(2)*u(8)
  qerr3 : Fcn  Expr=u(2)*u(5)-u(1)*u(6)+u(4)*u(7)+u(3)*u(8)
  qerr4 : Fcn  Expr=-u(1)*u(5)-u(2)*u(6)-u(3)*u(7)+u(4)*u(8)
  q_ac : Outport
  wires:
  Mux1/1 -> q_ac/1
  qerr4/1 -> Mux1/4
  qerr3/1 -> Mux1/3
  qerr2/1 -> Mux1/2
  qerr1/1 -> Mux1/1
  Mux/1 -> qerr4/1, qerr3/1, qerr2/1, qerr1/1
  q_ab/1 -> Mux/2
  q_bc/1 -> Mux/1

== matlab function single_sat_attitude/Attitude Determination/Attitude Determination/Generate reference vectors from Ephemeris and Magnetic Field Model/DecimalYearIncrement/MATLAB Function ==
  data: DecimalYear output; year input; month input; day input; hour input; minute input; second input
function DecimalYear = fcn(year,month,day,hour,minute,second)

for i=1:month-1
    if (month == 1 || month == 3 || month == 5 || month == 7 ...
             || month == 8 || month == 10 || month == 12)
         day= day+31;
    elseif (month == 2)
        if isLeapYear(year)
            day= day+29;
        else
            day= day+28;
        end
    else
        day= day+30;
    end
end
DecimalYear= year ...
            +day/(365+isLeapYear(year))   ...
            +hour/(365+isLeapYear(year))/24 ...
            +minute/(365+isLeapYear(year))/24/60 ...
            +second/(365+isLeapYear(year))/24/3600;
end
        
function logical=isLeapYear(year)
if (rem(year,4)==0)
    if (rem(year,100)==0)
        if (rem(year,400)==0)
            logical=1;
        else
            logical=0;
        end
    else
        logical=1;
    end
else
    logical=0;
end
end

== matlab function single_sat_attitude/Attitude Determination/Attitude Determination/Subsystem/MATLAB Function ==
  data: N_sun input; N_mag input; q_triad output; B_sun input; B_mag input
function q_triad = TRIAD(N_sun, N_mag, B_sun, B_mag)
%Based on time and the location of the spacecraft, the sun and magnetic 
%field vectors in the reference frame N are provided. Based on the sun
%sensor and magnetometer readings, the sun and magnetic field vectors are
%provided in the spacecraft's body frame B. This TRIAD algorithm is very
%straightforward and will not be used on the spacecraft, only for the
%sumulation. B/c the algorithm has the orientation of the same vectors in
%different reference frame, it is able to compute the rotation between
%those reference frames. The algorithm will fail if either of the reference
%vectors or observed vectors are parallel or anti parallel.

% Normalize all vectors (should be normalized already)
N_sun=N_sun/norm(N_sun);
B_sun=B_sun/norm(B_sun);
N_mag=N_mag/norm(N_mag);
B_mag=B_mag/norm(B_mag);

% Ensure all vectors have three components and vectors in the same frame
% are not parallel
if size(N_sun)~=[3 1]
    error('N_sun must be a 3-component column vector')
end

if size(B_sun)~=[3 1]
    error('B_sun must be a 3-component column vector')
end

if size(N_mag)~=[3 1]
    error('N_mag must be a 3-component column vector')
end

if size(B_mag)~=[3 1]
    error('B_mag must be a 3-component column vector')
end

if dot(N_sun,N_mag)==1
    error('Reference frame N vectors can not be parallel')
end

if dot(B_sun,B_mag)==1
    error('Body frame B vectors can not be parallel')
end

% Compute orthonogoal right-handed vectors of reference frame
v1=N_sun;
v2=cross(N_sun,N_mag)/norm(cross(N_sun,N_mag));
v3=cross(v1,v2);

% Compute orthonogoal right-handed vectors of body frame
w1=B_sun;
w2=cross(B_sun,B_mag)/norm(cross(B_sun,B_mag));
w3=cross(w1,w2);

DCM_be=w1(:)*v1(:)'+w3(:)*v3(:)'+w2(:)*v2(:)';
tr= DCM_be(1,1) + DCM_be(2,2) + DCM_be(3,3);
th= acos((tr-1)/2);
axis= 0.5/sin(th)*[DCM_be(2,3)-DCM_be(3,2);DCM_be(3,1)-DCM_be(1,3);DCM_be(1,2)-DCM_be(2,1)];
q_triad= [axis*sin(th/2);cos(th/2)];
%q_triad=dcm2quat(DCM_triad);
% q_temp=DCM_triad;
% q_triad=[q_temp(2) q_temp(3) q_temp(4) q_temp(1)];
end

== matlab function single_sat_attitude/Plant/Atm Torque and Force/pressureTorque ==
  data: pressure input; force output; unitvelocity input; areas input; unitnormals input; comtocops input; rss input; rds input; torque output
function [force,torque] = fcn(pressure,unitvelocity,areas,unitnormals,comtocops,rss,rds)
[force,torque] = pressureTorque(pressure,unitvelocity,areas,unitnormals,comtocops,rss,rds);

== matlab function single_sat_attitude/Plant/Reference Magfield /MATLAB Function ==
  data: t input; B output; x input
function B = fcn(t,x)
%sds
B= refMag(t,x);

== matlab function single_sat_attitude/Plant/Sun Torque and Force/pressureTorque ==
  data: pressure input; force output; unitvelocity input; areas input; unitnormals input; comtocops input; rss input; rds input; torque output
function [force,torque] = fcn(pressure,unitvelocity,areas,unitnormals,comtocops,rss,rds)
[force,torque] = pressureTorque(pressure,unitvelocity,areas,unitnormals,comtocops,rss,rds);

== stateflow chart single_sat_attitude/Mode Generator ==
  state Detumble
    entry: mode = 1;
    state High % Child State
      entry: y = 10;
    state Low % Child State
      entry: y = 1;
    (default) -> High % Child State
    Low % Child State -> High % Child State : after(1,sec)
    High % Child State -> Low % Child State : after(1,sec)
  state PowerON_RESET
    entry: mode= 1;
  state LargeAngleSlew
  (default) -> PowerON_RESET : {q_cmd_s= q_cmd;
      | q_body_s= q_body;
      | w_body_s= w_body;}
  PowerON_RESET -> Detumble [order 1] : [w_body >= w_dt]
  PowerON_RESET -> LargeAngleSlew [order 2]
  Detumble -> PowerON_RESET [order 1] : after(5,sec)
  Detumble -> LargeAngleSlew [order 2]
  data: q_body input; q_body_s local; q_cmd_s local; q_cmd input; w_body_s local; w_body input; mode output; w_dt parameter double
